simulink model "ssc_airvtol_elec_hybrid"  (R2021b)
settings: Solver=ode23t  StartTime=0.0  StopTime=FlightProfileLength  RelTol=1e-3  AbsTol=1e-3  EnableMultiTasking=on
PreLoadFcn:
  | ssc_airvtol_elec_default_params
PostLoadFcn:
  | warning('off','physmod:common:gl:sli:rtp:InvalidNonValueReference')
  | warning off Simulink:Engine:SortDiscontinuityInAlgLoop
model workspace (MATLAB code in the model file):
  | v0                 = 0; % Initial vehicle speed
  | wheel_radius = 0.15; % Wheel radius
  | k                   = 1e-2; % Motor losses (W/(N*M)^2)
  | t_torque        = 0.02; % Electric motor time constant
  | rpm0             = 2000; % Engine initial speed demand
undefined symbols (not defined in the file or in its folder): Based, engine_ref_speed, gen_torque_demand, Height, max_thrust, motor_ref_speed, propeller_num
libraries: fl_lib x115, nesl_utility x73, ee_lib x24, simulink x3, ssc_airvtol_elec_lib x2, sdl_lib x1, sh_lib x1
(part 3 of 3)

== system ssc_airvtol_elec_hybrid/Motor1/Torque Sensor ==
  PS-Simulink Converter : nesl_utility/PS-Simulink Converter  PhysicalDomain=network_engine_domain  SubClassName=ps_output  LeftPortType=input  RightPortType=output  PseudoPeriodic=off  Frequencies=[]  Unit=1  AffineConversion=off
      settings: SourceProductBaseCode=PW,SS
  Torque Sensor : fl_lib/Mechanical/Mechanical Sensors/Ideal Torque Sensor
      settings: SourceProductName=Foundation Library
  C : PMIOPort  Side=Right
  R : PMIOPort  Port=2  Side=Left
  trq : PMIOPort  Port=3  Side=Left
  tag scope: torque_mea1=global
  wires:
  PS-Simulink Converter/1 -> [torque_mea1]  "Measured Torque"
  connections:
  Torque Sensor/RConn2 -- trq/RConn1 -- PS-Simulink Converter/LConn1
  Torque Sensor/RConn1 -- C/RConn1
  Torque Sensor/LConn1 -- R/RConn1

== system ssc_airvtol_elec_hybrid/Motor2/Electrical Power ==
  " W to kW " : Gain  Gain=1/1000
  Current Sensor : fl_lib/Electrical/Electrical Sensors/Current Sensor
      settings: SourceProductName=Foundation Library
  PS Product : fl_lib/Physical Signals/Functions/PS Product
  PS-Simulink Converter : nesl_utility/PS-Simulink Converter  PhysicalDomain=network_engine_domain  SubClassName=ps_output  LeftPortType=input  RightPortType=output  PseudoPeriodic=off  Frequencies=[]  Unit=1  AffineConversion=off
      settings: SourceProductBaseCode=PW,SS
  PS-Simulink Converter3 : nesl_utility/PS-Simulink Converter  PhysicalDomain=network_engine_domain  SubClassName=ps_output  LeftPortType=input  RightPortType=output  PseudoPeriodic=off  Frequencies=[]  Unit=W  AffineConversion=off
      settings: SourceProductBaseCode=PW,SS
  Voltage Sensor : fl_lib/Electrical/Electrical Sensors/Voltage Sensor
      settings: SourceProductName=Foundation Library
  + : PMIOPort  Side=Left
  - : PMIOPort  Port=2  Side=Right
  0v : PMIOPort  Port=3  Side=Left
  tag scope: Current_Motor2=global, Pe_motor2=global
  wires:
  " W to kW "/1 -> [Pe_motor2]  "Motor Electrial Power"
  PS-Simulink Converter3/1 -> " W to kW "/1
  PS-Simulink Converter/1 -> [Current_Motor2]
  connections:
  PS Product/RConn1 -- PS-Simulink Converter3/LConn1
  Voltage Sensor/RConn1 -- PS Product/LConn2
  0v/RConn1 -- Voltage Sensor/RConn2
  Current Sensor/LConn1 -- +/RConn1
  Voltage Sensor/LConn1 -- Current Sensor/RConn2 -- -/RConn1
  Current Sensor/RConn1 -- PS-Simulink Converter/LConn1 -- PS Product/LConn1

== system ssc_airvtol_elec_hybrid/Motor2/Power ==
  " W to kW " : Gain  Gain=1/1000
  PS Product : fl_lib/Physical Signals/Functions/PS Product
  PS-Simulink Converter3 : nesl_utility/PS-Simulink Converter  PhysicalDomain=network_engine_domain  SubClassName=ps_output  LeftPortType=input  RightPortType=output  PseudoPeriodic=off  Frequencies=[]  Unit=W  AffineConversion=off
      settings: SourceProductBaseCode=PW,SS
  trq : PMIOPort  Side=Right
  w : PMIOPort  Port=2  Side=Right
  tag scope: Pm_motor2=global
  wires:
  " W to kW "/1 -> [Pm_motor2]  "Motor Mechanical Power"
  PS-Simulink Converter3/1 -> " W to kW "/1
  connections:
  PS Product/LConn1 -- trq/RConn1
  PS Product/LConn2 -- w/RConn1
  PS Product/RConn1 -- PS-Simulink Converter3/LConn1

== system ssc_airvtol_elec_hybrid/Motor2/RPM Sensor ==
  MRRef : fl_lib/Mechanical/Rotational Elements/Mechanical Rotational Reference
      settings: SourceProductName=Foundation Library
  Motion Sensor : fl_lib/Mechanical/Mechanical Sensors/Ideal Rotational Motion Sensor  wrap_angle=simscape.enum.onoff.off  offset=0 rad
      settings: SourceProductName=Foundation Library
  PS-Simulink Converter 2 : nesl_utility/PS-Simulink Converter  PhysicalDomain=network_engine_domain  SubClassName=ps_output  LeftPortType=input  RightPortType=output  PseudoPeriodic=off  Frequencies=[]  Unit=rpm  AffineConversion=off
      settings: SourceProductBaseCode=PW,SS
  R : PMIOPort  Side=Left
  rpm : Outport  VectorParamsAs1DForOutWhenUnconnected=off
  tag scope: motor2_rpm=global
  wires:
  PS-Simulink Converter 2/1 -> [motor2_rpm], rpm/1
  connections:
  R/RConn1 -- Motion Sensor/LConn1
  Motion Sensor/RConn1 -- MRRef/LConn1
  Motion Sensor/RConn2 -- PS-Simulink Converter 2/LConn1

== system ssc_airvtol_elec_hybrid/Motor2/Speed Controller ==
  rpm_ref : Inport
  rpm : Inport  Port=2
  20Hz Lowpass Filter : TransferFcn  Commented=through  Denominator=[1/(2*pi*20) 1]
  Ki : Gain  Gain=60
  Kp : Gain  Gain=60
  Limits [-40,40] : Integrator  LimitOutput=on  UpperSaturationLimit=40  LowerSaturationLimit=-40
  Sum : Sum  Inputs=-+|
  Sum1 : Sum  Inputs=++|
  "[-40,40]" : Saturate  UpperLimit=400  LowerLimit=-400
  T_ref : Outport  VectorParamsAs1DForOutWhenUnconnected=off
  wires:
  "[-40,40]"/1 -> T_ref/1
  20Hz Lowpass Filter/1 -> Sum/1
  Limits [-40,40]/1 -> Sum1/1
  Kp/1 -> Sum1/2
  Ki/1 -> Limits [-40,40]/1
  Sum/1 -> Kp/1, Ki/1
  Sum1/1 -> "[-40,40]"/1
  rpm/1 -> 20Hz Lowpass Filter/1
  rpm_ref/1 -> Sum/2

== system ssc_airvtol_elec_hybrid/Motor2/Torque Sensor ==
  PS-Simulink Converter : nesl_utility/PS-Simulink Converter  PhysicalDomain=network_engine_domain  SubClassName=ps_output  LeftPortType=input  RightPortType=output  PseudoPeriodic=off  Frequencies=[]  Unit=1  AffineConversion=off
      settings: SourceProductBaseCode=PW,SS
  Torque Sensor : fl_lib/Mechanical/Mechanical Sensors/Ideal Torque Sensor
      settings: SourceProductName=Foundation Library
  C : PMIOPort  Side=Right
  R : PMIOPort  Port=2  Side=Left
  trq : PMIOPort  Port=3  Side=Left
  tag scope: torque_mea2=global
  wires:
  PS-Simulink Converter/1 -> [torque_mea2]  "Measured Torque"
  connections:
  Torque Sensor/RConn2 -- trq/RConn1 -- PS-Simulink Converter/LConn1
  Torque Sensor/RConn1 -- C/RConn1
  Torque Sensor/LConn1 -- R/RConn1

== system ssc_airvtol_elec_hybrid/Motor3/Electrical Power ==
  " W to kW " : Gain  Gain=1/1000
  Current Sensor : fl_lib/Electrical/Electrical Sensors/Current Sensor
      settings: SourceProductName=Foundation Library
  PS Product : fl_lib/Physical Signals/Functions/PS Product
  PS-Simulink Converter : nesl_utility/PS-Simulink Converter  PhysicalDomain=network_engine_domain  SubClassName=ps_output  LeftPortType=input  RightPortType=output  PseudoPeriodic=off  Frequencies=[]  Unit=1  AffineConversion=off
      settings: SourceProductBaseCode=PW,SS
  PS-Simulink Converter3 : nesl_utility/PS-Simulink Converter  PhysicalDomain=network_engine_domain  SubClassName=ps_output  LeftPortType=input  RightPortType=output  PseudoPeriodic=off  Frequencies=[]  Unit=W  AffineConversion=off
      settings: SourceProductBaseCode=PW,SS
  Voltage Sensor : fl_lib/Electrical/Electrical Sensors/Voltage Sensor
      settings: SourceProductName=Foundation Library
  + : PMIOPort  Side=Left
  - : PMIOPort  Port=2  Side=Right
  0v : PMIOPort  Port=3  Side=Left
  tag scope: Current_Motor3=global, Pe_motor3=global
  wires:
  " W to kW "/1 -> [Pe_motor3]  "Motor Electrial Power"
  PS-Simulink Converter3/1 -> " W to kW "/1
  PS-Simulink Converter/1 -> [Current_Motor3]
  connections:
  PS Product/RConn1 -- PS-Simulink Converter3/LConn1
  Voltage Sensor/RConn1 -- PS Product/LConn2
  0v/RConn1 -- Voltage Sensor/RConn2
  Current Sensor/LConn1 -- +/RConn1
  Voltage Sensor/LConn1 -- Current Sensor/RConn2 -- -/RConn1
  Current Sensor/RConn1 -- PS-Simulink Converter/LConn1 -- PS Product/LConn1

== system ssc_airvtol_elec_hybrid/Motor3/Power ==
  " W to kW " : Gain  Gain=1/1000
  PS Product : fl_lib/Physical Signals/Functions/PS Product
  PS-Simulink Converter3 : nesl_utility/PS-Simulink Converter  PhysicalDomain=network_engine_domain  SubClassName=ps_output  LeftPortType=input  RightPortType=output  PseudoPeriodic=off  Frequencies=[]  Unit=W  AffineConversion=off
      settings: SourceProductBaseCode=PW,SS
  trq : PMIOPort  Side=Right
  w : PMIOPort  Port=2  Side=Right
  tag scope: Pm_motor3=global
  wires:
  " W to kW "/1 -> [Pm_motor3]  "Motor Mechanical Power"
  PS-Simulink Converter3/1 -> " W to kW "/1
  connections:
  PS Product/LConn1 -- trq/RConn1
  PS Product/LConn2 -- w/RConn1
  PS Product/RConn1 -- PS-Simulink Converter3/LConn1

== system ssc_airvtol_elec_hybrid/Motor3/RPM Sensor ==
  MRRef : fl_lib/Mechanical/Rotational Elements/Mechanical Rotational Reference
      settings: SourceProductName=Foundation Library
  Motion Sensor : fl_lib/Mechanical/Mechanical Sensors/Ideal Rotational Motion Sensor  wrap_angle=simscape.enum.onoff.off  offset=0 rad
      settings: SourceProductName=Foundation Library
  PS-Simulink Converter 2 : nesl_utility/PS-Simulink Converter  PhysicalDomain=network_engine_domain  SubClassName=ps_output  LeftPortType=input  RightPortType=output  PseudoPeriodic=off  Frequencies=[]  Unit=rpm  AffineConversion=off
      settings: SourceProductBaseCode=PW,SS
  R : PMIOPort  Side=Left
  rpm : Outport  VectorParamsAs1DForOutWhenUnconnected=off
  tag scope: motor3_rpm=global
  wires:
  PS-Simulink Converter 2/1 -> [motor3_rpm], rpm/1
  connections:
  R/RConn1 -- Motion Sensor/LConn1
  Motion Sensor/RConn1 -- MRRef/LConn1
  Motion Sensor/RConn2 -- PS-Simulink Converter 2/LConn1

== system ssc_airvtol_elec_hybrid/Motor3/Speed Controller ==
  rpm_ref : Inport
  rpm : Inport  Port=2
  20Hz Lowpass Filter : TransferFcn  Commented=through  Denominator=[1/(2*pi*20) 1]
  Ki : Gain  Gain=60
  Kp : Gain  Gain=60
  Limits [-40,40] : Integrator  LimitOutput=on  UpperSaturationLimit=40  LowerSaturationLimit=-40
  Sum : Sum  Inputs=-+|
  Sum1 : Sum  Inputs=++|
  "[-40,40]" : Saturate  UpperLimit=400  LowerLimit=-400
  T_ref : Outport  VectorParamsAs1DForOutWhenUnconnected=off
  wires:
  "[-40,40]"/1 -> T_ref/1
  20Hz Lowpass Filter/1 -> Sum/1
  Limits [-40,40]/1 -> Sum1/1
  Kp/1 -> Sum1/2
  Ki/1 -> Limits [-40,40]/1
  Sum/1 -> Kp/1, Ki/1
  Sum1/1 -> "[-40,40]"/1
  rpm/1 -> 20Hz Lowpass Filter/1
  rpm_ref/1 -> Sum/2

== system ssc_airvtol_elec_hybrid/Motor3/Torque Sensor ==
  PS-Simulink Converter : nesl_utility/PS-Simulink Converter  PhysicalDomain=network_engine_domain  SubClassName=ps_output  LeftPortType=input  RightPortType=output  PseudoPeriodic=off  Frequencies=[]  Unit=1  AffineConversion=off
      settings: SourceProductBaseCode=PW,SS
  Torque Sensor : fl_lib/Mechanical/Mechanical Sensors/Ideal Torque Sensor
      settings: SourceProductName=Foundation Library
  C : PMIOPort  Side=Right
  R : PMIOPort  Port=2  Side=Left
  trq : PMIOPort  Port=3  Side=Left
  tag scope: torque_mea3=global
  wires:
  PS-Simulink Converter/1 -> [torque_mea3]  "Measured Torque"
  connections:
  Torque Sensor/RConn2 -- trq/RConn1 -- PS-Simulink Converter/LConn1
  Torque Sensor/RConn1 -- C/RConn1
  Torque Sensor/LConn1 -- R/RConn1

== system ssc_airvtol_elec_hybrid/Motor4/Electrical Power ==
  " W to kW " : Gain  Gain=1/1000
  Current Sensor : fl_lib/Electrical/Electrical Sensors/Current Sensor
      settings: SourceProductName=Foundation Library
  PS Product : fl_lib/Physical Signals/Functions/PS Product
  PS-Simulink Converter : nesl_utility/PS-Simulink Converter  PhysicalDomain=network_engine_domain  SubClassName=ps_output  LeftPortType=input  RightPortType=output  PseudoPeriodic=off  Frequencies=[]  Unit=1  AffineConversion=off
      settings: SourceProductBaseCode=PW,SS
  PS-Simulink Converter3 : nesl_utility/PS-Simulink Converter  PhysicalDomain=network_engine_domain  SubClassName=ps_output  LeftPortType=input  RightPortType=output  PseudoPeriodic=off  Frequencies=[]  Unit=W  AffineConversion=off
      settings: SourceProductBaseCode=PW,SS
  Voltage Sensor : fl_lib/Electrical/Electrical Sensors/Voltage Sensor
      settings: SourceProductName=Foundation Library
  + : PMIOPort  Side=Left
  - : PMIOPort  Port=2  Side=Right
  0v : PMIOPort  Port=3  Side=Left
  tag scope: Current_Motor4=global, Pe_motor4=global
  wires:
  " W to kW "/1 -> [Pe_motor4]  "Motor Electrial Power"
  PS-Simulink Converter3/1 -> " W to kW "/1
  PS-Simulink Converter/1 -> [Current_Motor4]
  connections:
  PS Product/RConn1 -- PS-Simulink Converter3/LConn1
  Voltage Sensor/RConn1 -- PS Product/LConn2
  0v/RConn1 -- Voltage Sensor/RConn2
  Current Sensor/LConn1 -- +/RConn1
  Voltage Sensor/LConn1 -- Current Sensor/RConn2 -- -/RConn1
  Current Sensor/RConn1 -- PS-Simulink Converter/LConn1 -- PS Product/LConn1

== system ssc_airvtol_elec_hybrid/Motor4/Power ==
  " W to kW " : Gain  Gain=1/1000
  PS Product : fl_lib/Physical Signals/Functions/PS Product
  PS-Simulink Converter3 : nesl_utility/PS-Simulink Converter  PhysicalDomain=network_engine_domain  SubClassName=ps_output  LeftPortType=input  RightPortType=output  PseudoPeriodic=off  Frequencies=[]  Unit=W  AffineConversion=off
      settings: SourceProductBaseCode=PW,SS
  trq : PMIOPort  Side=Right
  w : PMIOPort  Port=2  Side=Right
  tag scope: Pm_motor4=global
  wires:
  " W to kW "/1 -> [Pm_motor4]  "Motor Mechanical Power"
  PS-Simulink Converter3/1 -> " W to kW "/1
  connections:
  PS Product/LConn1 -- trq/RConn1
  PS Product/LConn2 -- w/RConn1
  PS Product/RConn1 -- PS-Simulink Converter3/LConn1

== system ssc_airvtol_elec_hybrid/Motor4/RPM Sensor ==
  MRRef : fl_lib/Mechanical/Rotational Elements/Mechanical Rotational Reference
      settings: SourceProductName=Foundation Library
  Motion Sensor : fl_lib/Mechanical/Mechanical Sensors/Ideal Rotational Motion Sensor  wrap_angle=simscape.enum.onoff.off  offset=0 rad
      settings: SourceProductName=Foundation Library
  PS-Simulink Converter 2 : nesl_utility/PS-Simulink Converter  PhysicalDomain=network_engine_domain  SubClassName=ps_output  LeftPortType=input  RightPortType=output  PseudoPeriodic=off  Frequencies=[]  Unit=rpm  AffineConversion=off
      settings: SourceProductBaseCode=PW,SS
  R : PMIOPort  Side=Left
  rpm : Outport  VectorParamsAs1DForOutWhenUnconnected=off
  tag scope: motor4_rpm=global
  wires:
  PS-Simulink Converter 2/1 -> [motor4_rpm], rpm/1
  connections:
  R/RConn1 -- Motion Sensor/LConn1
  Motion Sensor/RConn1 -- MRRef/LConn1
  Motion Sensor/RConn2 -- PS-Simulink Converter 2/LConn1

== system ssc_airvtol_elec_hybrid/Motor4/Speed Controller ==
  rpm_ref : Inport
  rpm : Inport  Port=2
  20Hz Lowpass Filter : TransferFcn  Commented=through  Denominator=[1/(2*pi*20) 1]
  Ki : Gain  Gain=60
  Kp : Gain  Gain=60
  Limits [-40,40] : Integrator  LimitOutput=on  UpperSaturationLimit=40  LowerSaturationLimit=-40
  Sum : Sum  Inputs=-+|
  Sum1 : Sum  Inputs=++|
  "[-40,40]" : Saturate  UpperLimit=400  LowerLimit=-400
  T_ref : Outport  VectorParamsAs1DForOutWhenUnconnected=off
  wires:
  "[-40,40]"/1 -> T_ref/1
  20Hz Lowpass Filter/1 -> Sum/1
  Limits [-40,40]/1 -> Sum1/1
  Kp/1 -> Sum1/2
  Ki/1 -> Limits [-40,40]/1
  Sum/1 -> Kp/1, Ki/1
  Sum1/1 -> "[-40,40]"/1
  rpm/1 -> 20Hz Lowpass Filter/1
  rpm_ref/1 -> Sum/2

== system ssc_airvtol_elec_hybrid/Motor4/Torque Sensor ==
  PS-Simulink Converter : nesl_utility/PS-Simulink Converter  PhysicalDomain=network_engine_domain  SubClassName=ps_output  LeftPortType=input  RightPortType=output  PseudoPeriodic=off  Frequencies=[]  Unit=1  AffineConversion=off
      settings: SourceProductBaseCode=PW,SS
  Torque Sensor : fl_lib/Mechanical/Mechanical Sensors/Ideal Torque Sensor
      settings: SourceProductName=Foundation Library
  C : PMIOPort  Side=Right
  R : PMIOPort  Port=2  Side=Left
  trq : PMIOPort  Port=3  Side=Left
  tag scope: torque_mea4=global
  wires:
  PS-Simulink Converter/1 -> [torque_mea4]  "Measured Torque"
  connections:
  Torque Sensor/RConn2 -- trq/RConn1 -- PS-Simulink Converter/LConn1
  Torque Sensor/RConn1 -- C/RConn1
  Torque Sensor/LConn1 -- R/RConn1

== system ssc_airvtol_elec_hybrid/Motor5/Electrical Power ==
  " W to kW " : Gain  Gain=1/1000
  Current Sensor : fl_lib/Electrical/Electrical Sensors/Current Sensor
      settings: SourceProductName=Foundation Library
  PS Product : fl_lib/Physical Signals/Functions/PS Product
  PS-Simulink Converter : nesl_utility/PS-Simulink Converter  PhysicalDomain=network_engine_domain  SubClassName=ps_output  LeftPortType=input  RightPortType=output  PseudoPeriodic=off  Frequencies=[]  Unit=1  AffineConversion=off
      settings: SourceProductBaseCode=PW,SS
  PS-Simulink Converter3 : nesl_utility/PS-Simulink Converter  PhysicalDomain=network_engine_domain  SubClassName=ps_output  LeftPortType=input  RightPortType=output  PseudoPeriodic=off  Frequencies=[]  Unit=W  AffineConversion=off
      settings: SourceProductBaseCode=PW,SS
  Voltage Sensor : fl_lib/Electrical/Electrical Sensors/Voltage Sensor
      settings: SourceProductName=Foundation Library
  + : PMIOPort  Side=Left
  - : PMIOPort  Port=2  Side=Right
  0v : PMIOPort  Port=3  Side=Left
  tag scope: Current_Motor5=global, Pe_motor5=global
  wires:
  " W to kW "/1 -> [Pe_motor5]  "Motor Electrial Power"
  PS-Simulink Converter3/1 -> " W to kW "/1
  PS-Simulink Converter/1 -> [Current_Motor5]
  connections:
  PS Product/RConn1 -- PS-Simulink Converter3/LConn1
  Voltage Sensor/RConn1 -- PS Product/LConn2
  0v/RConn1 -- Voltage Sensor/RConn2
  Current Sensor/LConn1 -- +/RConn1
  Voltage Sensor/LConn1 -- Current Sensor/RConn2 -- -/RConn1
  Current Sensor/RConn1 -- PS-Simulink Converter/LConn1 -- PS Product/LConn1

== system ssc_airvtol_elec_hybrid/Motor5/Power ==
  " W to kW " : Gain  Gain=1/1000
  PS Product : fl_lib/Physical Signals/Functions/PS Product
  PS-Simulink Converter3 : nesl_utility/PS-Simulink Converter  PhysicalDomain=network_engine_domain  SubClassName=ps_output  LeftPortType=input  RightPortType=output  PseudoPeriodic=off  Frequencies=[]  Unit=W  AffineConversion=off
      settings: SourceProductBaseCode=PW,SS
  trq : PMIOPort  Side=Right
  w : PMIOPort  Port=2  Side=Right
  tag scope: Pm_motor5=global
  wires:
  " W to kW "/1 -> [Pm_motor5]  "Motor Mechanical Power"
  PS-Simulink Converter3/1 -> " W to kW "/1
  connections:
  PS Product/LConn1 -- trq/RConn1
  PS Product/LConn2 -- w/RConn1
  PS Product/RConn1 -- PS-Simulink Converter3/LConn1

== system ssc_airvtol_elec_hybrid/Motor5/RPM Sensor ==
  MRRef : fl_lib/Mechanical/Rotational Elements/Mechanical Rotational Reference
      settings: SourceProductName=Foundation Library
  Motion Sensor : fl_lib/Mechanical/Mechanical Sensors/Ideal Rotational Motion Sensor  wrap_angle=simscape.enum.onoff.off  offset=0 rad
      settings: SourceProductName=Foundation Library
  PS-Simulink Converter 2 : nesl_utility/PS-Simulink Converter  PhysicalDomain=network_engine_domain  SubClassName=ps_output  LeftPortType=input  RightPortType=output  PseudoPeriodic=off  Frequencies=[]  Unit=rpm  AffineConversion=off
      settings: SourceProductBaseCode=PW,SS
  R : PMIOPort  Side=Left
  rpm : Outport  VectorParamsAs1DForOutWhenUnconnected=off
  tag scope: motor5_rpm=global
  wires:
  PS-Simulink Converter 2/1 -> [motor5_rpm], rpm/1
  connections:
  R/RConn1 -- Motion Sensor/LConn1
  Motion Sensor/RConn1 -- MRRef/LConn1
  Motion Sensor/RConn2 -- PS-Simulink Converter 2/LConn1

== system ssc_airvtol_elec_hybrid/Motor5/Speed Controller ==
  rpm_ref : Inport
  rpm : Inport  Port=2
  20Hz Lowpass Filter : TransferFcn  Commented=through  Denominator=[1/(2*pi*20) 1]
  Ki : Gain  Gain=60
  Kp : Gain  Gain=60
  Limits [-40,40] : Integrator  LimitOutput=on  UpperSaturationLimit=40  LowerSaturationLimit=-40
  Sum : Sum  Inputs=-+|
  Sum1 : Sum  Inputs=++|
  "[-40,40]" : Saturate  UpperLimit=400  LowerLimit=-400
  T_ref : Outport  VectorParamsAs1DForOutWhenUnconnected=off
  wires:
  "[-40,40]"/1 -> T_ref/1
  20Hz Lowpass Filter/1 -> Sum/1
  Limits [-40,40]/1 -> Sum1/1
  Kp/1 -> Sum1/2
  Ki/1 -> Limits [-40,40]/1
  Sum/1 -> Kp/1, Ki/1
  Sum1/1 -> "[-40,40]"/1
  rpm/1 -> 20Hz Lowpass Filter/1
  rpm_ref/1 -> Sum/2

== system ssc_airvtol_elec_hybrid/Motor5/Torque Sensor ==
  PS-Simulink Converter : nesl_utility/PS-Simulink Converter  PhysicalDomain=network_engine_domain  SubClassName=ps_output  LeftPortType=input  RightPortType=output  PseudoPeriodic=off  Frequencies=[]  Unit=1  AffineConversion=off
      settings: SourceProductBaseCode=PW,SS
  Torque Sensor : fl_lib/Mechanical/Mechanical Sensors/Ideal Torque Sensor
      settings: SourceProductName=Foundation Library
  C : PMIOPort  Side=Right
  R : PMIOPort  Port=2  Side=Left
  trq : PMIOPort  Port=3  Side=Left
  tag scope: torque_mea5=global
  wires:
  PS-Simulink Converter/1 -> [torque_mea5]  "Measured Torque"
  connections:
  Torque Sensor/RConn2 -- trq/RConn1 -- PS-Simulink Converter/LConn1
  Torque Sensor/RConn1 -- C/RConn1
  Torque Sensor/LConn1 -- R/RConn1

== system ssc_airvtol_elec_hybrid/Motor6/Electrical Power ==
  " W to kW " : Gain  Gain=1/1000
  Current Sensor : fl_lib/Electrical/Electrical Sensors/Current Sensor
      settings: SourceProductName=Foundation Library
  PS Product : fl_lib/Physical Signals/Functions/PS Product
  PS-Simulink Converter : nesl_utility/PS-Simulink Converter  PhysicalDomain=network_engine_domain  SubClassName=ps_output  LeftPortType=input  RightPortType=output  PseudoPeriodic=off  Frequencies=[]  Unit=1  AffineConversion=off
      settings: SourceProductBaseCode=PW,SS
  PS-Simulink Converter3 : nesl_utility/PS-Simulink Converter  PhysicalDomain=network_engine_domain  SubClassName=ps_output  LeftPortType=input  RightPortType=output  PseudoPeriodic=off  Frequencies=[]  Unit=W  AffineConversion=off
      settings: SourceProductBaseCode=PW,SS
  Voltage Sensor : fl_lib/Electrical/Electrical Sensors/Voltage Sensor
      settings: SourceProductName=Foundation Library
  + : PMIOPort  Side=Left
  - : PMIOPort  Port=2  Side=Right
  0v : PMIOPort  Port=3  Side=Left
  tag scope: Current_Motor6=global, Pe_motor6=global
  wires:
  " W to kW "/1 -> [Pe_motor6]  "Motor Electrial Power"
  PS-Simulink Converter3/1 -> " W to kW "/1
  PS-Simulink Converter/1 -> [Current_Motor6]
  connections:
  PS Product/RConn1 -- PS-Simulink Converter3/LConn1
  Voltage Sensor/RConn1 -- PS Product/LConn2
  0v/RConn1 -- Voltage Sensor/RConn2
  Current Sensor/LConn1 -- +/RConn1
  Voltage Sensor/LConn1 -- Current Sensor/RConn2 -- -/RConn1
  Current Sensor/RConn1 -- PS-Simulink Converter/LConn1 -- PS Product/LConn1

== system ssc_airvtol_elec_hybrid/Motor6/Power ==
  " W to kW " : Gain  Gain=1/1000
  PS Product : fl_lib/Physical Signals/Functions/PS Product
  PS-Simulink Converter3 : nesl_utility/PS-Simulink Converter  PhysicalDomain=network_engine_domain  SubClassName=ps_output  LeftPortType=input  RightPortType=output  PseudoPeriodic=off  Frequencies=[]  Unit=W  AffineConversion=off
      settings: SourceProductBaseCode=PW,SS
  trq : PMIOPort  Side=Right
  w : PMIOPort  Port=2  Side=Right
  tag scope: Pm_motor6=global
  wires:
  " W to kW "/1 -> [Pm_motor6]  "Motor Mechanical Power"
  PS-Simulink Converter3/1 -> " W to kW "/1
  connections:
  PS Product/LConn1 -- trq/RConn1
  PS Product/LConn2 -- w/RConn1
  PS Product/RConn1 -- PS-Simulink Converter3/LConn1

== system ssc_airvtol_elec_hybrid/Motor6/RPM Sensor ==
  MRRef : fl_lib/Mechanical/Rotational Elements/Mechanical Rotational Reference
      settings: SourceProductName=Foundation Library
  Motion Sensor : fl_lib/Mechanical/Mechanical Sensors/Ideal Rotational Motion Sensor  wrap_angle=simscape.enum.onoff.off  offset=0 rad
      settings: SourceProductName=Foundation Library
  PS-Simulink Converter 2 : nesl_utility/PS-Simulink Converter  PhysicalDomain=network_engine_domain  SubClassName=ps_output  LeftPortType=input  RightPortType=output  PseudoPeriodic=off  Frequencies=[]  Unit=rpm  AffineConversion=off
      settings: SourceProductBaseCode=PW,SS
  R : PMIOPort  Side=Left
  rpm : Outport  VectorParamsAs1DForOutWhenUnconnected=off
  tag scope: motor6_rpm=global
  wires:
  PS-Simulink Converter 2/1 -> [motor6_rpm], rpm/1
  connections:
  R/RConn1 -- Motion Sensor/LConn1
  Motion Sensor/RConn1 -- MRRef/LConn1
  Motion Sensor/RConn2 -- PS-Simulink Converter 2/LConn1

== system ssc_airvtol_elec_hybrid/Motor6/Speed Controller ==
  rpm_ref : Inport
  rpm : Inport  Port=2
  20Hz Lowpass Filter : TransferFcn  Commented=through  Denominator=[1/(2*pi*20) 1]
  Ki : Gain  Gain=60
  Kp : Gain  Gain=60
  Limits [-40,40] : Integrator  LimitOutput=on  UpperSaturationLimit=40  LowerSaturationLimit=-40
  Sum : Sum  Inputs=-+|
  Sum1 : Sum  Inputs=++|
  "[-40,40]" : Saturate  UpperLimit=400  LowerLimit=-400
  T_ref : Outport  VectorParamsAs1DForOutWhenUnconnected=off
  wires:
  "[-40,40]"/1 -> T_ref/1
  20Hz Lowpass Filter/1 -> Sum/1
  Limits [-40,40]/1 -> Sum1/1
  Kp/1 -> Sum1/2
  Ki/1 -> Limits [-40,40]/1
  Sum/1 -> Kp/1, Ki/1
  Sum1/1 -> "[-40,40]"/1
  rpm/1 -> 20Hz Lowpass Filter/1
  rpm_ref/1 -> Sum/2

== system ssc_airvtol_elec_hybrid/Motor6/Torque Sensor ==
  PS-Simulink Converter : nesl_utility/PS-Simulink Converter  PhysicalDomain=network_engine_domain  SubClassName=ps_output  LeftPortType=input  RightPortType=output  PseudoPeriodic=off  Frequencies=[]  Unit=1  AffineConversion=off
      settings: SourceProductBaseCode=PW,SS
  Torque Sensor : fl_lib/Mechanical/Mechanical Sensors/Ideal Torque Sensor
      settings: SourceProductName=Foundation Library
  C : PMIOPort  Side=Right
  R : PMIOPort  Port=2  Side=Left
  trq : PMIOPort  Port=3  Side=Left
  tag scope: torque_mea6=global
  wires:
  PS-Simulink Converter/1 -> [torque_mea6]  "Measured Torque"
  connections:
  Torque Sensor/RConn2 -- trq/RConn1 -- PS-Simulink Converter/LConn1
  Torque Sensor/RConn1 -- C/RConn1
  Torque Sensor/LConn1 -- R/RConn1

== system ssc_airvtol_elec_hybrid/Motor7/Electrical Power ==
  " W to kW " : Gain  Gain=1/1000
  Current Sensor : fl_lib/Electrical/Electrical Sensors/Current Sensor
      settings: SourceProductName=Foundation Library
  PS Product : fl_lib/Physical Signals/Functions/PS Product
  PS-Simulink Converter : nesl_utility/PS-Simulink Converter  PhysicalDomain=network_engine_domain  SubClassName=ps_output  LeftPortType=input  RightPortType=output  PseudoPeriodic=off  Frequencies=[]  Unit=1  AffineConversion=off
      settings: SourceProductBaseCode=PW,SS
  PS-Simulink Converter3 : nesl_utility/PS-Simulink Converter  PhysicalDomain=network_engine_domain  SubClassName=ps_output  LeftPortType=input  RightPortType=output  PseudoPeriodic=off  Frequencies=[]  Unit=W  AffineConversion=off
      settings: SourceProductBaseCode=PW,SS
  Voltage Sensor : fl_lib/Electrical/Electrical Sensors/Voltage Sensor
      settings: SourceProductName=Foundation Library
  + : PMIOPort  Side=Left
  - : PMIOPort  Port=2  Side=Right
  0v : PMIOPort  Port=3  Side=Left
  tag scope: Current_Motor7=global, Pe_motor7=global
  wires:
  " W to kW "/1 -> [Pe_motor7]  "Motor Electrial Power"
  PS-Simulink Converter3/1 -> " W to kW "/1
  PS-Simulink Converter/1 -> [Current_Motor7]
  connections:
  PS Product/RConn1 -- PS-Simulink Converter3/LConn1
  Voltage Sensor/RConn1 -- PS Product/LConn2
  0v/RConn1 -- Voltage Sensor/RConn2
  Current Sensor/LConn1 -- +/RConn1
  Voltage Sensor/LConn1 -- Current Sensor/RConn2 -- -/RConn1
  Current Sensor/RConn1 -- PS-Simulink Converter/LConn1 -- PS Product/LConn1

== system ssc_airvtol_elec_hybrid/Motor7/Power ==
  " W to kW " : Gain  Gain=1/1000
  PS Product : fl_lib/Physical Signals/Functions/PS Product
  PS-Simulink Converter3 : nesl_utility/PS-Simulink Converter  PhysicalDomain=network_engine_domain  SubClassName=ps_output  LeftPortType=input  RightPortType=output  PseudoPeriodic=off  Frequencies=[]  Unit=W  AffineConversion=off
      settings: SourceProductBaseCode=PW,SS
  trq : PMIOPort  Side=Right
  w : PMIOPort  Port=2  Side=Right
  tag scope: Pm_motor7=global
  wires:
  " W to kW "/1 -> [Pm_motor7]  "Motor Mechanical Power"
  PS-Simulink Converter3/1 -> " W to kW "/1
  connections:
  PS Product/LConn1 -- trq/RConn1
  PS Product/LConn2 -- w/RConn1
  PS Product/RConn1 -- PS-Simulink Converter3/LConn1

== system ssc_airvtol_elec_hybrid/Motor7/RPM Sensor ==
  MRRef : fl_lib/Mechanical/Rotational Elements/Mechanical Rotational Reference
      settings: SourceProductName=Foundation Library
  Motion Sensor : fl_lib/Mechanical/Mechanical Sensors/Ideal Rotational Motion Sensor  wrap_angle=simscape.enum.onoff.off  offset=0 rad
      settings: SourceProductName=Foundation Library
  PS-Simulink Converter 2 : nesl_utility/PS-Simulink Converter  PhysicalDomain=network_engine_domain  SubClassName=ps_output  LeftPortType=input  RightPortType=output  PseudoPeriodic=off  Frequencies=[]  Unit=rpm  AffineConversion=off
      settings: SourceProductBaseCode=PW,SS
  R : PMIOPort  Side=Left
  rpm : Outport  VectorParamsAs1DForOutWhenUnconnected=off
  tag scope: motor7_rpm=global
  wires:
  PS-Simulink Converter 2/1 -> [motor7_rpm], rpm/1
  connections:
  R/RConn1 -- Motion Sensor/LConn1
  Motion Sensor/RConn1 -- MRRef/LConn1
  Motion Sensor/RConn2 -- PS-Simulink Converter 2/LConn1

== system ssc_airvtol_elec_hybrid/Motor7/Speed Controller ==
  rpm_ref : Inport
  rpm : Inport  Port=2
  20Hz Lowpass Filter : TransferFcn  Commented=through  Denominator=[1/(2*pi*20) 1]
  Ki : Gain  Gain=60
  Kp : Gain  Gain=60
  Limits [-40,40] : Integrator  LimitOutput=on  UpperSaturationLimit=40  LowerSaturationLimit=-40
  Sum : Sum  Inputs=-+|
  Sum1 : Sum  Inputs=++|
  "[-40,40]" : Saturate  UpperLimit=400  LowerLimit=-400
  T_ref : Outport  VectorParamsAs1DForOutWhenUnconnected=off
  wires:
  "[-40,40]"/1 -> T_ref/1
  20Hz Lowpass Filter/1 -> Sum/1
  Limits [-40,40]/1 -> Sum1/1
  Kp/1 -> Sum1/2
  Ki/1 -> Limits [-40,40]/1
  Sum/1 -> Kp/1, Ki/1
  Sum1/1 -> "[-40,40]"/1
  rpm/1 -> 20Hz Lowpass Filter/1
  rpm_ref/1 -> Sum/2

== system ssc_airvtol_elec_hybrid/Motor7/Torque Sensor ==
  PS-Simulink Converter : nesl_utility/PS-Simulink Converter  PhysicalDomain=network_engine_domain  SubClassName=ps_output  LeftPortType=input  RightPortType=output  PseudoPeriodic=off  Frequencies=[]  Unit=1  AffineConversion=off
      settings: SourceProductBaseCode=PW,SS
  Torque Sensor : fl_lib/Mechanical/Mechanical Sensors/Ideal Torque Sensor
      settings: SourceProductName=Foundation Library
  C : PMIOPort  Side=Right
  R : PMIOPort  Port=2  Side=Left
  trq : PMIOPort  Port=3  Side=Left
  tag scope: torque_mea7=global
  wires:
  PS-Simulink Converter/1 -> [torque_mea7]  "Measured Torque"
  connections:
  Torque Sensor/RConn2 -- trq/RConn1 -- PS-Simulink Converter/LConn1
  Torque Sensor/RConn1 -- C/RConn1
  Torque Sensor/LConn1 -- R/RConn1

== system ssc_airvtol_elec_hybrid/Motor8/Electrical Power ==
  " W to kW " : Gain  Gain=1/1000
  Current Sensor : fl_lib/Electrical/Electrical Sensors/Current Sensor
      settings: SourceProductName=Foundation Library
  PS Product : fl_lib/Physical Signals/Functions/PS Product
  PS-Simulink Converter : nesl_utility/PS-Simulink Converter  PhysicalDomain=network_engine_domain  SubClassName=ps_output  LeftPortType=input  RightPortType=output  PseudoPeriodic=off  Frequencies=[]  Unit=1  AffineConversion=off
      settings: SourceProductBaseCode=PW,SS
  PS-Simulink Converter3 : nesl_utility/PS-Simulink Converter  PhysicalDomain=network_engine_domain  SubClassName=ps_output  LeftPortType=input  RightPortType=output  PseudoPeriodic=off  Frequencies=[]  Unit=W  AffineConversion=off
      settings: SourceProductBaseCode=PW,SS
  Voltage Sensor : fl_lib/Electrical/Electrical Sensors/Voltage Sensor
      settings: SourceProductName=Foundation Library
  + : PMIOPort  Side=Left
  - : PMIOPort  Port=2  Side=Right
  0v : PMIOPort  Port=3  Side=Left
  tag scope: Current_Motor8=global, Pe_motor8=global
  wires:
  " W to kW "/1 -> [Pe_motor8]  "Motor Electrial Power"
  PS-Simulink Converter3/1 -> " W to kW "/1
  PS-Simulink Converter/1 -> [Current_Motor8]
  connections:
  PS Product/RConn1 -- PS-Simulink Converter3/LConn1
  Voltage Sensor/RConn1 -- PS Product/LConn2
  0v/RConn1 -- Voltage Sensor/RConn2
  Current Sensor/LConn1 -- +/RConn1
  Voltage Sensor/LConn1 -- Current Sensor/RConn2 -- -/RConn1
  Current Sensor/RConn1 -- PS-Simulink Converter/LConn1 -- PS Product/LConn1

== system ssc_airvtol_elec_hybrid/Motor8/Power ==
  " W to kW " : Gain  Gain=1/1000
  PS Product : fl_lib/Physical Signals/Functions/PS Product
  PS-Simulink Converter3 : nesl_utility/PS-Simulink Converter  PhysicalDomain=network_engine_domain  SubClassName=ps_output  LeftPortType=input  RightPortType=output  PseudoPeriodic=off  Frequencies=[]  Unit=W  AffineConversion=off
      settings: SourceProductBaseCode=PW,SS
  trq : PMIOPort  Side=Right
  w : PMIOPort  Port=2  Side=Right
  tag scope: Pm_motor8=global
  wires:
  " W to kW "/1 -> [Pm_motor8]  "Motor Mechanical Power"
  PS-Simulink Converter3/1 -> " W to kW "/1
  connections:
  PS Product/LConn1 -- trq/RConn1
  PS Product/LConn2 -- w/RConn1
  PS Product/RConn1 -- PS-Simulink Converter3/LConn1

== system ssc_airvtol_elec_hybrid/Motor8/RPM Sensor ==
  MRRef : fl_lib/Mechanical/Rotational Elements/Mechanical Rotational Reference
      settings: SourceProductName=Foundation Library
  Motion Sensor : fl_lib/Mechanical/Mechanical Sensors/Ideal Rotational Motion Sensor  wrap_angle=simscape.enum.onoff.off  offset=0 rad
      settings: SourceProductName=Foundation Library
  PS-Simulink Converter 2 : nesl_utility/PS-Simulink Converter  PhysicalDomain=network_engine_domain  SubClassName=ps_output  LeftPortType=input  RightPortType=output  PseudoPeriodic=off  Frequencies=[]  Unit=rpm  AffineConversion=off
      settings: SourceProductBaseCode=PW,SS
  R : PMIOPort  Side=Left
  rpm : Outport  VectorParamsAs1DForOutWhenUnconnected=off
  tag scope: motor8_rpm=global
  wires:
  PS-Simulink Converter 2/1 -> [motor8_rpm], rpm/1
  connections:
  R/RConn1 -- Motion Sensor/LConn1
  Motion Sensor/RConn1 -- MRRef/LConn1
  Motion Sensor/RConn2 -- PS-Simulink Converter 2/LConn1

== system ssc_airvtol_elec_hybrid/Motor8/Speed Controller ==
  rpm_ref : Inport
  rpm : Inport  Port=2
  20Hz Lowpass Filter : TransferFcn  Commented=through  Denominator=[1/(2*pi*20) 1]
  Ki : Gain  Gain=60
  Kp : Gain  Gain=60
  Limits [-40,40] : Integrator  LimitOutput=on  UpperSaturationLimit=40  LowerSaturationLimit=-40
  Sum : Sum  Inputs=-+|
  Sum1 : Sum  Inputs=++|
  "[-40,40]" : Saturate  UpperLimit=400  LowerLimit=-400
  T_ref : Outport  VectorParamsAs1DForOutWhenUnconnected=off
  wires:
  "[-40,40]"/1 -> T_ref/1
  20Hz Lowpass Filter/1 -> Sum/1
  Limits [-40,40]/1 -> Sum1/1
  Kp/1 -> Sum1/2
  Ki/1 -> Limits [-40,40]/1
  Sum/1 -> Kp/1, Ki/1
  Sum1/1 -> "[-40,40]"/1
  rpm/1 -> 20Hz Lowpass Filter/1
  rpm_ref/1 -> Sum/2

== system ssc_airvtol_elec_hybrid/Motor8/Torque Sensor ==
  PS-Simulink Converter : nesl_utility/PS-Simulink Converter  PhysicalDomain=network_engine_domain  SubClassName=ps_output  LeftPortType=input  RightPortType=output  PseudoPeriodic=off  Frequencies=[]  Unit=1  AffineConversion=off
      settings: SourceProductBaseCode=PW,SS
  Torque Sensor : fl_lib/Mechanical/Mechanical Sensors/Ideal Torque Sensor
      settings: SourceProductName=Foundation Library
  C : PMIOPort  Side=Right
  R : PMIOPort  Port=2  Side=Left
  trq : PMIOPort  Port=3  Side=Left
  tag scope: torque_mea8=global
  wires:
  PS-Simulink Converter/1 -> [torque_mea8]  "Measured Torque"
  connections:
  Torque Sensor/RConn2 -- trq/RConn1 -- PS-Simulink Converter/LConn1
  Torque Sensor/RConn1 -- C/RConn1
  Torque Sensor/LConn1 -- R/RConn1

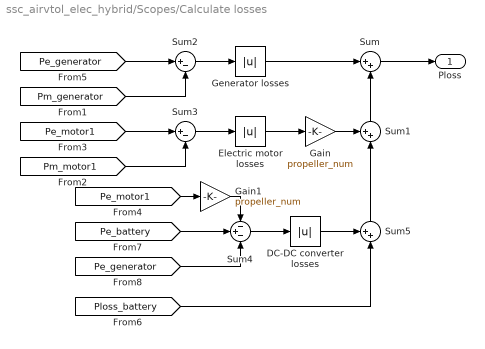
== system ssc_airvtol_elec_hybrid/Scopes/Calculate losses ==
  " Electric motor losses" : Abs  SaturateOnIntegerOverflow=on
  DC-DC converter losses : Abs  SaturateOnIntegerOverflow=on
  Gain : Gain  Gain=propeller_num
  Gain1 : Gain  Gain=propeller_num
  Generator losses : Abs  SaturateOnIntegerOverflow=on
  Sum : Sum  Inputs=|++
  Sum1 : Sum  Inputs=++|
  Sum2 : Sum  Inputs=|+-
  Sum3 : Sum  Inputs=|+-
  Sum4 : Sum  Inputs=-+-
  Sum5 : Sum  Inputs=++|
  Ploss : Outport  VectorParamsAs1DForOutWhenUnconnected=off
  wires:
  [Ploss_battery] -> Sum5/2
  DC-DC converter losses/1 -> Sum5/1
  " Electric motor losses"/1 -> Gain/1
  [Pe_generator] -> Sum4/3
  [Pe_motor1] -> Gain1/1
  [Pe_battery] -> Sum4/2
  Sum5/1 -> Sum1/2
  Sum4/1 -> DC-DC converter losses/1
  Sum3/1 -> " Electric motor losses"/1
  [Pm_motor1] -> Sum3/2
  [Pe_motor1] -> Sum3/1
  Generator losses/1 -> Sum/1
  Sum2/1 -> Generator losses/1
  [Pm_generator] -> Sum2/2
  [Pe_generator] -> Sum2/1
  Sum/1 -> Ploss/1
  Sum1/1 -> Sum/2
  Gain/1 -> Sum1/1
  Gain1/1 -> Sum4/1

== system ssc_airvtol_elec_hybrid/Sensing/Calculations ==
  " W to kW " : Gain  Gain=1/1000
  I^2 : fl_lib/Physical Signals/Functions/PS Product
  PS-Simulink Converter : nesl_utility/PS-Simulink Converter  PhysicalDomain=network_engine_domain  SubClassName=ps_output  LeftPortType=input  RightPortType=output  PseudoPeriodic=off  Frequencies=[]  Unit=W  AffineConversion=off
      settings: SourceProductBaseCode=PW,SS
  PS-Simulink Converter4 : nesl_utility/PS-Simulink Converter  PhysicalDomain=network_engine_domain  SubClassName=ps_output  LeftPortType=input  RightPortType=output  PseudoPeriodic=off  Frequencies=[]  Unit=W  AffineConversion=off
      settings: SourceProductBaseCode=PW,SS
  Power : fl_lib/Physical Signals/Functions/PS Product
  R : fl_lib/Physical Signals/Functions/PS Gain  gain=0.05 Ohm
  W to kW : Gain  Gain=1/1000
  I : PMIOPort  Side=Left
  V : PMIOPort  Port=2  Side=Left
  tag scope: Pe_battery=global, Ploss_battery=global
  wires:
  " W to kW "/1 -> [Ploss_battery]
  PS-Simulink Converter4/1 -> " W to kW "/1
  W to kW/1 -> [Pe_battery]  "Battery Power"
  PS-Simulink Converter/1 -> W to kW/1  "Battery power"
  connections:
  R/RConn1 -- PS-Simulink Converter4/LConn1
  I^2/RConn1 -- R/LConn1
  I^2/LConn1 -- I^2/LConn2 -- I/RConn1 -- Power/LConn2
  V/RConn1 -- Power/LConn1
  Power/RConn1 -- PS-Simulink Converter/LConn1
